simulink model "Copy_5_of_baseModel"  (R2019a)
settings: Solver=ode1  StartTime=0.0  StopTime=2.5  FixedStep=Ts_Power  RelTol=1e-3
PostLoadFcn:
  | %% Init for wind PnO models - global system parameters
  | OVERRIDE_SSN_MEMORY_LIMIT=1;
  | Ts=50e-6;
  | % Ts=50e-10;
  | Ts_Power=Ts;
  | Ts_Control=2*Ts;
  | freq = 50;
  | Fnom=freq;
  | Vac=400e3;
InitFcn:
  | %% Init for wind PnO models - global system parameters
  | OVERRIDE_SSN_MEMORY_LIMIT=1;
  | Ts=50e-6;
  | % Ts=50e-10;
  | Ts_Power=Ts;
  | Ts_Control=2*Ts;
  | freq = 50;
  | Fnom=freq;
  | Vac=225e3;
values from neighbouring files (symbols this model uses):
  ohl_posCap = (0.01e-006)*12    (= 1.2e-07)    [variable.m]
  ohl_posInd = (1.15e-3)/12    (= 9.58333333333e-05)    [variable.m]
  ohl_posR = 0.069/12    (= 0.00575)    [variable.m]
  ohl_zeroCap = (0.004e-006)*12    (= 4.8e-08)    [variable.m]
  ohl_zeroInd = (2.86e-3)/12    (= 0.000238333333333)    [variable.m]
  ohl_zeroR = 0.1725/12    (= 0.014375)    [variable.m]
  sub_posCap = sub_posCap*6    (= 9.6e-07)    [variable.m]
  sub_posInd = sub_posInd/6    (= 0.000233333333333)    [variable.m]
  sub_posR = sub_posR/6    (= 0.006)    [variable.m]
  sub_zeroCap = sub_zeroCap*6    (= 3.84e-07)    [variable.m]
  sub_zeroInd = sub_zeroInd/6    (= 0.000583333333333)    [variable.m]
  sub_zeroR = sub_zeroR/6    (= 0.015)    [variable.m]
  transfo_L1 = 0.05999374    [variable.m]
  transfo_L2 = 0.05999374    [variable.m]
  transfo_R1 = 0.000866667    [variable.m]
  transfo_R2 = 0.00086667    [variable.m]
undefined symbols (not defined in the file or in its folder): D1, D11, Delta, den, DiscIntNeverNeededParam, dx, find_system, gcbh, num, out_Buses, out_WindFarms, sps_rtmsupport
libraries: powerlib x200, simulink x96, powerlib_meascontrol x96, elements x52, eeSinusoidalMeasurement x51, simulink_extras x42, spsVIMeasurementModel x36, eePowerMeasurement x16
(part 12 of 24)

== system Copy_5_of_baseModel/SM_WT1/Impedance Element 1/Impedance Relay Scheme/Fault C-A Measurement ==
  C-A : Inport
  <V : Inport  Port=2
  Complex to Real-Imag : ComplexToRealImag
  Impedance Module : Product  Inputs=*/  SaturateOnIntegerOverflow=on  RndMeth=Zero  InputSameDT=on  OutDataTypeStr=Inherit: Same as first input
  Mux{,1..4} (5 alike) : Mux  Inputs=2
  Voltage Current : Demux  Outputs=2
  Zone 1 : Subsystem  mask(Zone){Xr=ZoneImpedance(1)*sin(LineAngle*pi/180), Rr=ZoneImpedance(1)*cos(LineAngle*pi/180), Td=ZoneTime(1)}
      mask prompts: Xr "Reactance reach [ohm]"; Rr "Resistance reach [ohm]"; Td "Time delay [s]"
  Zone 2 : Subsystem  mask(Zone){Xr=ZoneImpedance(2)*sin(LineAngle*pi/180), Rr=ZoneImpedance(2)*cos(LineAngle*pi/180), Td=ZoneTime(2)}
      mask prompts: Xr "Reactance reach [ohm]"; Rr "Resistance reach [ohm]"; Td "Time delay [s]"
  Zone 3 : Subsystem  mask(Zone){Xr=ZoneImpedance(3)*sin(LineAngle*pi/180), Rr=ZoneImpedance(3)*cos(LineAngle*pi/180), Td=ZoneTime(3)}
      mask prompts: Xr "Reactance reach [ohm]"; Rr "Resistance reach [ohm]"; Td "Time delay [s]"
  Zone 4 : Subsystem  mask(Zone){Xr=ZoneImpedance(4)*sin(LineAngle*pi/180), Rr=ZoneImpedance(4)*cos(LineAngle*pi/180), Td=ZoneTime(4)}
      mask prompts: Xr "Reactance reach [ohm]"; Rr "Resistance reach [ohm]"; Td "Time delay [s]"
  Zone1Z : Terminator
  Zone2Z : Terminator
  Zone3Z : Terminator
  Zone4Z : Terminator
  Zone1 : Outport  InitialOutput=0  VectorParamsAs1DForOutWhenUnconnected=on
  Zone2 : Outport  Port=2  InitialOutput=0  VectorParamsAs1DForOutWhenUnconnected=on
  Zone3 : Outport  Port=3  InitialOutput=0  VectorParamsAs1DForOutWhenUnconnected=on
  Zone4 : Outport  Port=4  InitialOutput=0  VectorParamsAs1DForOutWhenUnconnected=on
  wires:
  Voltage Current/2 -> Impedance Module/2
  Voltage Current/1 -> Impedance Module/1
  Impedance Module/1 -> Complex to Real-Imag/1
  Mux4/1 -> Zone4Z/1
  Mux3/1 -> Zone3Z/1
  Mux2/1 -> Zone2Z/1
  Mux1/1 -> Zone1Z/1
  <V/1 -> Zone 4/2(<V), Zone 3/2(<V), Zone 2/2(<V), Zone 1/2(<V)
  Complex to Real-Imag/2 -> Mux/2
  Complex to Real-Imag/1 -> Mux/1
  Zone 4/1(TRIP) -> Zone4/1
  Zone 3/1(TRIP) -> Zone3/1
  Zone 2/1(TRIP) -> Zone2/1
  Zone 4/3(Zr) -> Mux4/2
  Zone 4/2(Zm) -> Mux4/1
  Zone 3/3(Zr) -> Mux3/2
  Zone 3/2(Zm) -> Mux3/1
  Zone 2/3(Zr) -> Mux2/2
  Zone 2/2(Zm) -> Mux2/1
  Zone 1/3(Zr) -> Mux1/2
  Zone 1/2(Zm) -> Mux1/1
  Zone 1/1(TRIP) -> Zone1/1
  Mux/1 -> Zone 2/1(Z), Zone 4/1(Z), Zone 3/1(Z), Zone 1/1(Z)
  C-A/1 -> Voltage Current/1

== system Copy_5_of_baseModel/SM_WT1/Impedance Element 1/Impedance Relay Scheme/Fault C-G Measurement ==
  C-G : Inport
  <V : Inport  Port=2
  Complex to Real-Imag : ComplexToRealImag
  Impedance Module : Product  Inputs=*/  SaturateOnIntegerOverflow=on  RndMeth=Zero  InputSameDT=on  OutDataTypeStr=Inherit: Same as first input
  Mux{,1..4} (5 alike) : Mux  Inputs=2
  Voltage Current : Demux  Outputs=2
  Zone 1 : Subsystem  mask(Zone){Xr=ZoneImpedance(1)*sin(LineAngle*pi/180), Rr=ZoneImpedance(1)*cos(LineAngle*pi/180), Td=ZoneTime(1)}
      mask prompts: Xr "Reactance reach [ohm]"; Rr "Resistance reach [ohm]"; Td "Time delay [s]"
  Zone 2 : Subsystem  mask(Zone){Xr=ZoneImpedance(2)*sin(LineAngle*pi/180), Rr=ZoneImpedance(2)*cos(LineAngle*pi/180), Td=ZoneTime(2)}
      mask prompts: Xr "Reactance reach [ohm]"; Rr "Resistance reach [ohm]"; Td "Time delay [s]"
  Zone 3 : Subsystem  mask(Zone){Xr=ZoneImpedance(3)*sin(LineAngle*pi/180), Rr=ZoneImpedance(3)*cos(LineAngle*pi/180), Td=ZoneTime(3)}
      mask prompts: Xr "Reactance reach [ohm]"; Rr "Resistance reach [ohm]"; Td "Time delay [s]"
  Zone 4 : Subsystem  mask(Zone){Xr=ZoneImpedance(4)*sin(LineAngle*pi/180), Rr=ZoneImpedance(4)*cos(LineAngle*pi/180), Td=ZoneTime(4)}
      mask prompts: Xr "Reactance reach [ohm]"; Rr "Resistance reach [ohm]"; Td "Time delay [s]"
  Zone1Z : Terminator
  Zone2Z : Terminator
  Zone3Z : Terminator
  Zone4Z : Terminator
  Zone1 : Outport  InitialOutput=0  VectorParamsAs1DForOutWhenUnconnected=on
  Zone2 : Outport  Port=2  InitialOutput=0  VectorParamsAs1DForOutWhenUnconnected=on
  Zone3 : Outport  Port=3  InitialOutput=0  VectorParamsAs1DForOutWhenUnconnected=on
  Zone4 : Outport  Port=4  InitialOutput=0  VectorParamsAs1DForOutWhenUnconnected=on
  wires:
  Voltage Current/2 -> Impedance Module/2
  Voltage Current/1 -> Impedance Module/1
  Impedance Module/1 -> Complex to Real-Imag/1
  Mux4/1 -> Zone4Z/1
  Mux3/1 -> Zone3Z/1
  Mux2/1 -> Zone2Z/1
  Mux1/1 -> Zone1Z/1
  <V/1 -> Zone 4/2(<V), Zone 3/2(<V), Zone 2/2(<V), Zone 1/2(<V)
  Complex to Real-Imag/2 -> Mux/2
  Complex to Real-Imag/1 -> Mux/1
  Zone 4/1(TRIP) -> Zone4/1
  Zone 3/1(TRIP) -> Zone3/1
  Zone 2/1(TRIP) -> Zone2/1
  Zone 4/3(Zr) -> Mux4/2
  Zone 4/2(Zm) -> Mux4/1
  Zone 3/3(Zr) -> Mux3/2
  Zone 3/2(Zm) -> Mux3/1
  Zone 2/3(Zr) -> Mux2/2
  Zone 2/2(Zm) -> Mux2/1
  Zone 1/3(Zr) -> Mux1/2
  Zone 1/2(Zm) -> Mux1/1
  Zone 1/1(TRIP) -> Zone1/1
  Mux/1 -> Zone 2/1(Z), Zone 4/1(Z), Zone 3/1(Z), Zone 1/1(Z)
  C-G/1 -> Voltage Current/1

== system Copy_5_of_baseModel/SM_WT1/Impedance Element 1/Impedance Relay Scheme/Logic Matrix ==
  note: Impedance Relay - Logic Signal Matrix
  A-G : Inport
  B-G : Inport  Port=2
  C-G : Inport  Port=3
  B-C : Inport  Port=4
  C-A : Inport  Port=5
  A-B-C : Inport  Port=6
  A : Logic  Operator=OR  Inputs=3
  A-B-C1 : Logic  Operator=OR  Inputs=4
  "A-G1 " : Logic  Operator=OR  Inputs=4
  B : Logic  Operator=OR  Inputs=3
  B-C1 : Logic  Operator=OR  Inputs=4
  B-G1 : Logic  Operator=OR  Inputs=4
  C : Logic  Operator=OR  Inputs=4
  C-A1 : Logic  Operator=OR  Inputs=4
  C-G1 : Logic  Operator=OR  Inputs=4
  Demux{,1..5} (6 alike) : Demux
  G : Logic  Operator=OR  Inputs=3
  Mux5 : Mux
  zone{1..4} (4 alike) : Logic  Operator=OR  Inputs=6
  " Zone1" : Outport  InitialOutput=0  VectorParamsAs1DForOutWhenUnconnected=on
  " Zone2" : Outport  Port=2  InitialOutput=0  VectorParamsAs1DForOutWhenUnconnected=on
  " Zone3" : Outport  Port=3  InitialOutput=0  VectorParamsAs1DForOutWhenUnconnected=on
  " Zone4" : Outport  Port=4  InitialOutput=0  VectorParamsAs1DForOutWhenUnconnected=on
  Fault Type : Outport  Port=5  InitialOutput=0  VectorParamsAs1DForOutWhenUnconnected=on
  wires:
  G/1 -> Mux5/4
  C/1 -> Mux5/3
  B/1 -> Mux5/2
  A/1 -> Mux5/1
  B-G1/1 -> G/2, B/1
  C-G1/1 -> G/1, C/1
  B-C1/1 -> C/2, B/2
  A-B-C1/1 -> B/3, A/3, C/4
  C-A1/1 -> A/2, C/3
  "A-G1 "/1 -> G/3, A/1
  Demux5/4 -> A-B-C1/4, zone4/6
  Demux5/3 -> A-B-C1/3, zone3/6
  Demux5/2 -> A-B-C1/2, zone2/6
  Demux5/1 -> A-B-C1/1, zone1/6
  Demux4/4 -> C-A1/4, zone4/5
  Demux4/3 -> C-A1/3, zone3/5
  Demux4/2 -> C-A1/2, zone2/5
  Demux4/1 -> C-A1/1, zone1/5
  Demux3/4 -> B-C1/4, zone4/4
  Demux3/3 -> B-C1/3, zone3/4
  Demux3/2 -> B-C1/2, zone2/4
  Demux3/1 -> B-C1/1, zone1/4
  Demux2/4 -> C-G1/4, zone4/3
  Demux2/3 -> C-G1/3, zone3/3
  Demux2/2 -> C-G1/2, zone2/3
  Demux2/1 -> C-G1/1, zone1/3
  Demux1/4 -> B-G1/4, zone4/2
  Demux1/3 -> B-G1/3, zone3/2
  Demux1/2 -> B-G1/2, zone2/2
  Demux1/1 -> B-G1/1, zone1/2
  Demux/4 -> "A-G1 "/4, zone4/1
  Demux/3 -> "A-G1 "/3, zone3/1
  Demux/2 -> "A-G1 "/2, zone2/1
  Demux/1 -> "A-G1 "/1, zone1/1
  A-G/1 -> Demux/1
  B-G/1 -> Demux1/1
  A-B-C/1 -> Demux5/1
  C-A/1 -> Demux4/1
  B-C/1 -> Demux3/1
  C-G/1 -> Demux2/1
  Mux5/1 -> Fault Type/1
  zone1/1 -> " Zone1"/1
  zone2/1 -> " Zone2"/1
  zone4/1 -> " Zone4"/1
  zone3/1 -> " Zone3"/1

== system Copy_5_of_baseModel/SM_WT1/Impedance Element 1/Impedance Relay Scheme/Tripping Logic ==
  note: Impedance Relay - Tripping Logic
  zone1 : Inport
  zone2 : Inport  Port=2
  zone3 : Inport  Port=3
  zone4 : Inport  Port=4
  <V : Inport  Port=5
  Add{,1..3} (4 alike) : Sum
  Constant : Constant  Value=2
  Mux : Mux  Inputs=5
  Mux6 : Mux
  ZM1 + ZM2*t2 + ZM3*t3 + ZM4*t4 : Logic  Operator=OR  Inputs=4
  x2 : Gain  Gain=2  SaturateOnIntegerOverflow=on  OutDataTypeStr=Inherit: Same as input  ParamDataTypeStr=Inherit: Same as input
  x3 : Gain  Gain=3  SaturateOnIntegerOverflow=on  OutDataTypeStr=Inherit: Same as input  ParamDataTypeStr=Inherit: Same as input
  x4 : Gain  Gain=4  SaturateOnIntegerOverflow=on  OutDataTypeStr=Inherit: Same as input  ParamDataTypeStr=Inherit: Same as input
  TRIP : Outport  InitialOutput=0  VectorParamsAs1DForOutWhenUnconnected=on
  Logic Signals : Outport  Port=2  InitialOutput=0  VectorParamsAs1DForOutWhenUnconnected=on
  Fault Zone : Outport  Port=3  InitialOutput=0  VectorParamsAs1DForOutWhenUnconnected=on
  wires:
  Mux6/1 -> Fault Zone/1
  x3/1 -> Add2/2
  x4/1 -> Add3/2
  x2/1 -> Add1/2
  Constant/1 -> x4/1, x3/1, x2/1, Add/2
  Add3/1 -> Mux/5
  Add2/1 -> Mux/4
  Add1/1 -> Mux/3
  Add/1 -> Mux/2
  zone4/1 -> Mux6/4, Add3/1, ZM1 + ZM2*t2 + ZM3*t3 + ZM4*t4/4
  zone3/1 -> Mux6/3, Add2/1, ZM1 + ZM2*t2 + ZM3*t3 + ZM4*t4/3
  zone2/1 -> Add1/1, Mux6/2, ZM1 + ZM2*t2 + ZM3*t3 + ZM4*t4/2
  zone1/1 -> Mux6/1, Add/1, ZM1 + ZM2*t2 + ZM3*t3 + ZM4*t4/1
  ZM1 + ZM2*t2 + ZM3*t3 + ZM4*t4/1 -> TRIP/1
  Mux/1 -> Logic Signals/1
  <V/1 -> Mux/1

== system Copy_5_of_baseModel/SM_WT1/Impedance Element 1/Impedance Relay Scheme/Undervoltage ==
  "Vabc  " : Inport
  Abs : Abs
  Abs1 : Abs
  Abs2 : Abs
  Demux2 : Demux  Outputs=3
  Logical Operator : Logic  Operator=OR  Inputs=3
  Relational Operator : RelationalOperator  Operator=<  RndMeth=Nearest  InputSameDT=on
  Relational Operator1 : RelationalOperator  Operator=<  RndMeth=Nearest  InputSameDT=on
  Relational Operator2 : RelationalOperator  Operator=<  RndMeth=Nearest  InputSameDT=on
  underV Threshold : Constant  Value=underV
  <V : Outport  InitialOutput=0  VectorParamsAs1DForOutWhenUnconnected=on
  wires:
  Demux2/3 -> Abs2/1
  Demux2/2 -> Abs1/1
  Abs1/1 -> Relational Operator2/1
  Abs2/1 -> Relational Operator1/1
  Demux2/1 -> Abs/1
  Abs/1 -> Relational Operator/1
  Relational Operator1/1 -> Logical Operator/3
  Relational Operator/1 -> Logical Operator/1
  Relational Operator2/1 -> Logical Operator/2
  Logical Operator/1 -> <V/1
  underV Threshold/1 -> Relational Operator1/2, Relational Operator2/2, Relational Operator/2
  "Vabc  "/1 -> Demux2/1

== system Copy_5_of_baseModel/SM_WT1/Impedance Element 2/Impedance Relay Scheme/Analog filtering, signal conditioning ==
  note: Acquisition Block- analog filtering,
      | signal conditioning, sampling.
  Vin : Inport
  Iin : Inport  Port=2
  CURRENTS : Subsystem
  Mux{1..4} (4 alike) : Mux  Inputs=3
  VOLTAGES : Subsystem
  Vf : Outport  InitialOutput=0  VectorParamsAs1DForOutWhenUnconnected=on
  If : Outport  Port=2  InitialOutput=0  VectorParamsAs1DForOutWhenUnconnected=on
  If0 : Outport  Port=3  InitialOutput=0  VectorParamsAs1DForOutWhenUnconnected=on
  vf : Outport  Port=4  InitialOutput=0  VectorParamsAs1DForOutWhenUnconnected=on
  if : Outport  Port=5  InitialOutput=0  VectorParamsAs1DForOutWhenUnconnected=on
  wires:
  CURRENTS/4(k0I0f) -> If0/1
  Mux4/1 -> if/1
  Mux3/1 -> If/1
  CURRENTS/7(icf) -> Mux4/3
  CURRENTS/6(ibf) -> Mux4/2
  CURRENTS/5(iaf) -> Mux4/1
  CURRENTS/3(ICf) -> Mux3/3
  CURRENTS/2(IBf) -> Mux3/2
  CURRENTS/1(IAf) -> Mux3/1
  Iin/1 -> CURRENTS/1(Iabc)
  Mux2/1 -> vf/1
  VOLTAGES/6(vcf) -> Mux2/3
  VOLTAGES/5(vbf) -> Mux2/2
  VOLTAGES/4(vaf) -> Mux2/1
  VOLTAGES/3(VCf) -> Mux1/3
  VOLTAGES/2(VBf) -> Mux1/2
  VOLTAGES/1(VAf) -> Mux1/1
  Vin/1 -> VOLTAGES/1(Vabc)
  Mux1/1 -> Vf/1

== system Copy_5_of_baseModel/SM_WT1/Impedance Element 2/Impedance Relay Scheme/Combination of Voltages and Currents into 6 pairs (for each type of fault) ==
  note: Voltage and current combination block
  Vf : Inport
  If : Inport  Port=2
  If0 : Inport  Port=3
  "Currents Ia, Ib, Ic, kIo" : Demux  Outputs=3
  Ia+kIo : Sum  SaturateOnIntegerOverflow=on  InputSameDT=on  OutDataTypeStr=Inherit: Same as first input
  Ia-Ib : Sum  Inputs=+-  SaturateOnIntegerOverflow=on  InputSameDT=on  OutDataTypeStr=Inherit: Same as first input
  Ib+kIo : Sum  SaturateOnIntegerOverflow=on  InputSameDT=on  OutDataTypeStr=Inherit: Same as first input
  Ib-Ic : Sum  Inputs=+-  SaturateOnIntegerOverflow=on  InputSameDT=on  OutDataTypeStr=Inherit: Same as first input
  Ic+kIo : Sum  SaturateOnIntegerOverflow=on  InputSameDT=on  OutDataTypeStr=Inherit: Same as first input
  Ic-Ia : Sum  Inputs=+-  SaturateOnIntegerOverflow=on  InputSameDT=on  OutDataTypeStr=Inherit: Same as first input
  Mux{10..15} (6 alike) : Mux  Inputs=2
  Va-Vb : Sum  Inputs=+-  SaturateOnIntegerOverflow=on  InputSameDT=on  OutDataTypeStr=Inherit: Same as first input
  Vb-Vc : Sum  Inputs=+-  SaturateOnIntegerOverflow=on  InputSameDT=on  OutDataTypeStr=Inherit: Same as first input
  Vc-Va : Sum  Inputs=+-  SaturateOnIntegerOverflow=on  InputSameDT=on  OutDataTypeStr=Inherit: Same as first input
  "Voltages Va,Vb, Vc" : Demux  Outputs=3
  "Volt, Curr A-G" : Outport  InitialOutput=0  VectorParamsAs1DForOutWhenUnconnected=on
  "Volt, Curr B-G" : Outport  Port=2  InitialOutput=0  VectorParamsAs1DForOutWhenUnconnected=on
  "Volt, Curr C-G" : Outport  Port=3  InitialOutput=0  VectorParamsAs1DForOutWhenUnconnected=on
  "Volt, Curr B-C,B-C-G" : Outport  Port=4  InitialOutput=0  VectorParamsAs1DForOutWhenUnconnected=on
  "Volt, Curr C-A,C-A-G" : Outport  Port=5  InitialOutput=0  VectorParamsAs1DForOutWhenUnconnected=on
  "Volt, Curr A-B,A-B-C-G" : Outport  Port=6  InitialOutput=0  VectorParamsAs1DForOutWhenUnconnected=on
  wires:
  If0/1 -> Ib+kIo/2, Ia+kIo/2, Ic+kIo/2
  Mux13/1 -> "Volt, Curr B-C,B-C-G"/1
  Vb-Vc/1 -> Mux13/1
  Ib-Ic/1 -> Mux13/2
  Mux12/1 -> "Volt, Curr C-G"/1
  Ic+kIo/1 -> Mux12/2
  If/1 -> "Currents Ia, Ib, Ic, kIo"/1
  "Voltages Va,Vb, Vc"/3 -> Vc-Va/1, Vb-Vc/2, Mux12/1
  "Voltages Va,Vb, Vc"/2 -> Vb-Vc/1, Mux11/1, Va-Vb/2
  "Voltages Va,Vb, Vc"/1 -> Va-Vb/1, Mux10/1, Vc-Va/2
  Vf/1 -> "Voltages Va,Vb, Vc"/1
  Mux15/1 -> "Volt, Curr A-B,A-B-C-G"/1
  Mux14/1 -> "Volt, Curr C-A,C-A-G"/1
  Vc-Va/1 -> Mux14/1
  Mux11/1 -> "Volt, Curr B-G"/1
  Mux10/1 -> "Volt, Curr A-G"/1
  Ia+kIo/1 -> Mux10/2
  Ib+kIo/1 -> Mux11/2
  Ic-Ia/1 -> Mux14/2
  Va-Vb/1 -> Mux15/1
  Ia-Ib/1 -> Mux15/2
  "Currents Ia, Ib, Ic, kIo"/2 -> Ia-Ib/2, Ib-Ic/1, Ib+kIo/1
  "Currents Ia, Ib, Ic, kIo"/3 -> Ic-Ia/1, Ib-Ic/2, Ic+kIo/1
  "Currents Ia, Ib, Ic, kIo"/1 -> Ia-Ib/1, Ic-Ia/2, Ia+kIo/1

== system Copy_5_of_baseModel/SM_WT1/Impedance Element 2/Impedance Relay Scheme/Fault A-B-C Measurement ==
  A-B-C : Inport
  <V : Inport  Port=2
  Complex to Real-Imag : ComplexToRealImag
  Impedance Module : Product  Inputs=*/  SaturateOnIntegerOverflow=on  RndMeth=Zero  InputSameDT=on  OutDataTypeStr=Inherit: Same as first input
  Mux{,1..4} (5 alike) : Mux  Inputs=2
  Voltage Current : Demux  Outputs=2
  Zone 1 : Subsystem  mask(Zone){Xr=ZoneImpedance(1)*sin(LineAngle*pi/180), Rr=ZoneImpedance(1)*cos(LineAngle*pi/180), Td=ZoneTime(1)}
      mask prompts: Xr "Reactance reach [ohm]"; Rr "Resistance reach [ohm]"; Td "Time delay [s]"
  Zone 2 : Subsystem  mask(Zone){Xr=ZoneImpedance(2)*sin(LineAngle*pi/180), Rr=ZoneImpedance(2)*cos(LineAngle*pi/180), Td=ZoneTime(2)}
      mask prompts: Xr "Reactance reach [ohm]"; Rr "Resistance reach [ohm]"; Td "Time delay [s]"
  Zone 3 : Subsystem  mask(Zone){Xr=ZoneImpedance(3)*sin(LineAngle*pi/180), Rr=ZoneImpedance(3)*cos(LineAngle*pi/180), Td=ZoneTime(3)}
      mask prompts: Xr "Reactance reach [ohm]"; Rr "Resistance reach [ohm]"; Td "Time delay [s]"
  Zone 4 : Subsystem  mask(Zone){Xr=ZoneImpedance(4)*sin(LineAngle*pi/180), Rr=ZoneImpedance(4)*cos(LineAngle*pi/180), Td=ZoneTime(4)}
      mask prompts: Xr "Reactance reach [ohm]"; Rr "Resistance reach [ohm]"; Td "Time delay [s]"
  Zone1Z : Terminator
  Zone2Z : Terminator
  Zone3Z : Terminator
  Zone4Z : Terminator
  Zone1 : Outport  InitialOutput=0  VectorParamsAs1DForOutWhenUnconnected=on
  Zone2 : Outport  Port=2  InitialOutput=0  VectorParamsAs1DForOutWhenUnconnected=on
  Zone3 : Outport  Port=3  InitialOutput=0  VectorParamsAs1DForOutWhenUnconnected=on
  Zone4 : Outport  Port=4  InitialOutput=0  VectorParamsAs1DForOutWhenUnconnected=on
  wires:
  A-B-C/1 -> Voltage Current/1
  Mux/1 -> Zone 1/1(Z), Zone 3/1(Z), Zone 4/1(Z), Zone 2/1(Z)
  Zone 1/1(TRIP) -> Zone1/1
  Zone 1/2(Zm) -> Mux1/1
  Zone 1/3(Zr) -> Mux1/2
  Zone 2/2(Zm) -> Mux2/1
  Zone 2/3(Zr) -> Mux2/2
  Zone 3/2(Zm) -> Mux3/1
  Zone 3/3(Zr) -> Mux3/2
  Zone 4/2(Zm) -> Mux4/1
  Zone 4/3(Zr) -> Mux4/2
  Zone 2/1(TRIP) -> Zone2/1
  Zone 3/1(TRIP) -> Zone3/1
  Zone 4/1(TRIP) -> Zone4/1
  Complex to Real-Imag/1 -> Mux/1
  Complex to Real-Imag/2 -> Mux/2
  <V/1 -> Zone 1/2(<V), Zone 2/2(<V), Zone 3/2(<V), Zone 4/2(<V)
  Mux1/1 -> Zone1Z/1
  Mux2/1 -> Zone2Z/1
  Mux3/1 -> Zone3Z/1
  Mux4/1 -> Zone4Z/1
  Impedance Module/1 -> Complex to Real-Imag/1
  Voltage Current/1 -> Impedance Module/1
  Voltage Current/2 -> Impedance Module/2

== system Copy_5_of_baseModel/SM_WT1/Impedance Element 2/Impedance Relay Scheme/Fault A-G Measurement ==
  A-G : Inport
  <V : Inport  Port=2
  Complex to Real-Imag : ComplexToRealImag
  Impedance Module : Product  Inputs=*/  SaturateOnIntegerOverflow=on  RndMeth=Zero  InputSameDT=on  OutDataTypeStr=Inherit: Same as first input
  Mux{,1..4} (5 alike) : Mux  Inputs=2
  Voltage Current : Demux  Outputs=2
  Zone 1 : Subsystem  mask(Zone){Xr=ZoneImpedance(1)*sin(LineAngle*pi/180), Rr=ZoneImpedance(1)*cos(LineAngle*pi/180), Td=ZoneTime(1)}
      mask prompts: Xr "Reactance reach [ohm]"; Rr "Resistance reach [ohm]"; Td "Time delay [s]"
  Zone 2 : Subsystem  mask(Zone){Xr=ZoneImpedance(2)*sin(LineAngle*pi/180), Rr=ZoneImpedance(2)*cos(LineAngle*pi/180), Td=ZoneTime(2)}
      mask prompts: Xr "Reactance reach [ohm]"; Rr "Resistance reach [ohm]"; Td "Time delay [s]"
  Zone 3 : Subsystem  mask(Zone){Xr=ZoneImpedance(3)*sin(LineAngle*pi/180), Rr=ZoneImpedance(3)*cos(LineAngle*pi/180), Td=ZoneTime(3)}
      mask prompts: Xr "Reactance reach [ohm]"; Rr "Resistance reach [ohm]"; Td "Time delay [s]"
  Zone 4 : Subsystem  mask(Zone){Xr=ZoneImpedance(4)*sin(LineAngle*pi/180), Rr=ZoneImpedance(4)*cos(LineAngle*pi/180), Td=ZoneTime(4)}
      mask prompts: Xr "Reactance reach [ohm]"; Rr "Resistance reach [ohm]"; Td "Time delay [s]"
  Zone1Z : Terminator
  Zone2Z : Terminator
  Zone3Z : Terminator
  Zone4Z : Terminator
  Zone1 : Outport  InitialOutput=0  VectorParamsAs1DForOutWhenUnconnected=on
  Zone2 : Outport  Port=2  InitialOutput=0  VectorParamsAs1DForOutWhenUnconnected=on
  Zone3 : Outport  Port=3  InitialOutput=0  VectorParamsAs1DForOutWhenUnconnected=on
  Zone4 : Outport  Port=4  InitialOutput=0  VectorParamsAs1DForOutWhenUnconnected=on
  wires:
  Voltage Current/2 -> Impedance Module/2
  Voltage Current/1 -> Impedance Module/1
  Impedance Module/1 -> Complex to Real-Imag/1
  Mux4/1 -> Zone4Z/1
  Mux3/1 -> Zone3Z/1
  Mux2/1 -> Zone2Z/1
  Mux1/1 -> Zone1Z/1
  <V/1 -> Zone 4/2(<V), Zone 3/2(<V), Zone 2/2(<V), Zone 1/2(<V)
  Complex to Real-Imag/2 -> Mux/2
  Complex to Real-Imag/1 -> Mux/1
  Zone 4/1(TRIP) -> Zone4/1
  Zone 3/1(TRIP) -> Zone3/1
  Zone 2/1(TRIP) -> Zone2/1
  Zone 4/3(Zr) -> Mux4/2
  Zone 4/2(Zm) -> Mux4/1
  Zone 3/3(Zr) -> Mux3/2
  Zone 3/2(Zm) -> Mux3/1
  Zone 2/3(Zr) -> Mux2/2
  Zone 2/2(Zm) -> Mux2/1
  Zone 1/3(Zr) -> Mux1/2
  Zone 1/2(Zm) -> Mux1/1
  Zone 1/1(TRIP) -> Zone1/1
  Mux/1 -> Zone 2/1(Z), Zone 4/1(Z), Zone 3/1(Z), Zone 1/1(Z)
  A-G/1 -> Voltage Current/1

== system Copy_5_of_baseModel/SM_WT1/Impedance Element 2/Impedance Relay Scheme/Fault B-C Measurement ==
  B-C : Inport
  <V : Inport  Port=2
  Complex to Real-Imag : ComplexToRealImag
  Impedance Module : Product  Inputs=*/  SaturateOnIntegerOverflow=on  RndMeth=Zero  InputSameDT=on  OutDataTypeStr=Inherit: Same as first input
  Mux{,1..4} (5 alike) : Mux  Inputs=2
  Voltage Current : Demux  Outputs=2
  Zone 1 : Subsystem  mask(Zone){Xr=ZoneImpedance(1)*sin(LineAngle*pi/180), Rr=ZoneImpedance(1)*cos(LineAngle*pi/180), Td=ZoneTime(1)}
      mask prompts: Xr "Reactance reach [ohm]"; Rr "Resistance reach [ohm]"; Td "Time delay [s]"
  Zone 2 : Subsystem  mask(Zone){Xr=ZoneImpedance(2)*sin(LineAngle*pi/180), Rr=ZoneImpedance(2)*cos(LineAngle*pi/180), Td=ZoneTime(2)}
      mask prompts: Xr "Reactance reach [ohm]"; Rr "Resistance reach [ohm]"; Td "Time delay [s]"
  Zone 3 : Subsystem  mask(Zone){Xr=ZoneImpedance(3)*sin(LineAngle*pi/180), Rr=ZoneImpedance(3)*cos(LineAngle*pi/180), Td=ZoneTime(3)}
      mask prompts: Xr "Reactance reach [ohm]"; Rr "Resistance reach [ohm]"; Td "Time delay [s]"
  Zone 4 : Subsystem  mask(Zone){Xr=ZoneImpedance(4)*sin(LineAngle*pi/180), Rr=ZoneImpedance(4)*cos(LineAngle*pi/180), Td=ZoneTime(4)}
      mask prompts: Xr "Reactance reach [ohm]"; Rr "Resistance reach [ohm]"; Td "Time delay [s]"
  Zone1Z : Terminator
  Zone2Z : Terminator
  Zone3Z : Terminator
  Zone4Z : Terminator
  Zone1 : Outport  InitialOutput=0  VectorParamsAs1DForOutWhenUnconnected=on
  Zone2 : Outport  Port=2  InitialOutput=0  VectorParamsAs1DForOutWhenUnconnected=on
  Zone3 : Outport  Port=3  InitialOutput=0  VectorParamsAs1DForOutWhenUnconnected=on
  Zone4 : Outport  Port=4  InitialOutput=0  VectorParamsAs1DForOutWhenUnconnected=on
  wires:
  B-C/1 -> Voltage Current/1
  Mux/1 -> Zone 1/1(Z), Zone 3/1(Z), Zone 4/1(Z), Zone 2/1(Z)
  Zone 1/1(TRIP) -> Zone1/1
  Zone 1/2(Zm) -> Mux1/1
  Zone 1/3(Zr) -> Mux1/2
  Zone 2/2(Zm) -> Mux2/1
  Zone 2/3(Zr) -> Mux2/2
  Zone 3/2(Zm) -> Mux3/1
  Zone 3/3(Zr) -> Mux3/2
  Zone 4/2(Zm) -> Mux4/1
  Zone 4/3(Zr) -> Mux4/2
  Zone 2/1(TRIP) -> Zone2/1
  Zone 3/1(TRIP) -> Zone3/1
  Zone 4/1(TRIP) -> Zone4/1
  Complex to Real-Imag/1 -> Mux/1
  Complex to Real-Imag/2 -> Mux/2
  <V/1 -> Zone 1/2(<V), Zone 2/2(<V), Zone 3/2(<V), Zone 4/2(<V)
  Mux1/1 -> Zone1Z/1
  Mux2/1 -> Zone2Z/1
  Mux3/1 -> Zone3Z/1
  Mux4/1 -> Zone4Z/1
  Impedance Module/1 -> Complex to Real-Imag/1
  Voltage Current/1 -> Impedance Module/1
  Voltage Current/2 -> Impedance Module/2

== system Copy_5_of_baseModel/SM_WT1/Impedance Element 2/Impedance Relay Scheme/Fault B-G Measurement ==
  B-G : Inport
  <V : Inport  Port=2
  Complex to Real-Imag : ComplexToRealImag
  Impedance Module : Product  Inputs=*/  SaturateOnIntegerOverflow=on  RndMeth=Zero  InputSameDT=on  OutDataTypeStr=Inherit: Same as first input
  Mux{,1..4} (5 alike) : Mux  Inputs=2
  Voltage Current : Demux  Outputs=2
  Zone 1 : Subsystem  mask(Zone){Xr=ZoneImpedance(1)*sin(LineAngle*pi/180), Rr=ZoneImpedance(1)*cos(LineAngle*pi/180), Td=ZoneTime(1)}
      mask prompts: Xr "Reactance reach [ohm]"; Rr "Resistance reach [ohm]"; Td "Time delay [s]"
  Zone 2 : Subsystem  mask(Zone){Xr=ZoneImpedance(2)*sin(LineAngle*pi/180), Rr=ZoneImpedance(2)*cos(LineAngle*pi/180), Td=ZoneTime(2)}
      mask prompts: Xr "Reactance reach [ohm]"; Rr "Resistance reach [ohm]"; Td "Time delay [s]"
  Zone 3 : Subsystem  mask(Zone){Xr=ZoneImpedance(3)*sin(LineAngle*pi/180), Rr=ZoneImpedance(3)*cos(LineAngle*pi/180), Td=ZoneTime(3)}
      mask prompts: Xr "Reactance reach [ohm]"; Rr "Resistance reach [ohm]"; Td "Time delay [s]"
  Zone 4 : Subsystem  mask(Zone){Xr=ZoneImpedance(4)*sin(LineAngle*pi/180), Rr=ZoneImpedance(4)*cos(LineAngle*pi/180), Td=ZoneTime(4)}
      mask prompts: Xr "Reactance reach [ohm]"; Rr "Resistance reach [ohm]"; Td "Time delay [s]"
  Zone1Z : Terminator
  Zone2Z : Terminator
  Zone3Z : Terminator
  Zone4Z : Terminator
  Zone1 : Outport  InitialOutput=0  VectorParamsAs1DForOutWhenUnconnected=on
  Zone2 : Outport  Port=2  InitialOutput=0  VectorParamsAs1DForOutWhenUnconnected=on
  Zone3 : Outport  Port=3  InitialOutput=0  VectorParamsAs1DForOutWhenUnconnected=on
  Zone4 : Outport  Port=4  InitialOutput=0  VectorParamsAs1DForOutWhenUnconnected=on
  wires:
  B-G/1 -> Voltage Current/1
  Mux/1 -> Zone 1/1(Z), Zone 3/1(Z), Zone 4/1(Z), Zone 2/1(Z)
  Zone 1/1(TRIP) -> Zone1/1
  Zone 1/2(Zm) -> Mux1/1
  Zone 1/3(Zr) -> Mux1/2
  Zone 2/2(Zm) -> Mux2/1
  Zone 2/3(Zr) -> Mux2/2
  Zone 3/2(Zm) -> Mux3/1
  Zone 3/3(Zr) -> Mux3/2
  Zone 4/2(Zm) -> Mux4/1
  Zone 4/3(Zr) -> Mux4/2
  Zone 2/1(TRIP) -> Zone2/1
  Zone 3/1(TRIP) -> Zone3/1
  Zone 4/1(TRIP) -> Zone4/1
  Complex to Real-Imag/1 -> Mux/1
  Complex to Real-Imag/2 -> Mux/2
  <V/1 -> Zone 1/2(<V), Zone 2/2(<V), Zone 3/2(<V), Zone 4/2(<V)
  Mux1/1 -> Zone1Z/1
  Mux2/1 -> Zone2Z/1
  Mux3/1 -> Zone3Z/1
  Mux4/1 -> Zone4Z/1
  Impedance Module/1 -> Complex to Real-Imag/1
  Voltage Current/1 -> Impedance Module/1
  Voltage Current/2 -> Impedance Module/2

== system Copy_5_of_baseModel/SM_WT1/Impedance Element 2/Impedance Relay Scheme/Fault C-A Measurement ==
  C-A : Inport
  <V : Inport  Port=2
  Complex to Real-Imag : ComplexToRealImag
  Impedance Module : Product  Inputs=*/  SaturateOnIntegerOverflow=on  RndMeth=Zero  InputSameDT=on  OutDataTypeStr=Inherit: Same as first input
  Mux{,1..4} (5 alike) : Mux  Inputs=2
  Voltage Current : Demux  Outputs=2
  Zone 1 : Subsystem  mask(Zone){Xr=ZoneImpedance(1)*sin(LineAngle*pi/180), Rr=ZoneImpedance(1)*cos(LineAngle*pi/180), Td=ZoneTime(1)}
      mask prompts: Xr "Reactance reach [ohm]"; Rr "Resistance reach [ohm]"; Td "Time delay [s]"
  Zone 2 : Subsystem  mask(Zone){Xr=ZoneImpedance(2)*sin(LineAngle*pi/180), Rr=ZoneImpedance(2)*cos(LineAngle*pi/180), Td=ZoneTime(2)}
      mask prompts: Xr "Reactance reach [ohm]"; Rr "Resistance reach [ohm]"; Td "Time delay [s]"
  Zone 3 : Subsystem  mask(Zone){Xr=ZoneImpedance(3)*sin(LineAngle*pi/180), Rr=ZoneImpedance(3)*cos(LineAngle*pi/180), Td=ZoneTime(3)}
      mask prompts: Xr "Reactance reach [ohm]"; Rr "Resistance reach [ohm]"; Td "Time delay [s]"
  Zone 4 : Subsystem  mask(Zone){Xr=ZoneImpedance(4)*sin(LineAngle*pi/180), Rr=ZoneImpedance(4)*cos(LineAngle*pi/180), Td=ZoneTime(4)}
      mask prompts: Xr "Reactance reach [ohm]"; Rr "Resistance reach [ohm]"; Td "Time delay [s]"
  Zone1Z : Terminator
  Zone2Z : Terminator
  Zone3Z : Terminator
  Zone4Z : Terminator
  Zone1 : Outport  InitialOutput=0  VectorParamsAs1DForOutWhenUnconnected=on
  Zone2 : Outport  Port=2  InitialOutput=0  VectorParamsAs1DForOutWhenUnconnected=on
  Zone3 : Outport  Port=3  InitialOutput=0  VectorParamsAs1DForOutWhenUnconnected=on
  Zone4 : Outport  Port=4  InitialOutput=0  VectorParamsAs1DForOutWhenUnconnected=on
  wires:
  Voltage Current/2 -> Impedance Module/2
  Voltage Current/1 -> Impedance Module/1
  Impedance Module/1 -> Complex to Real-Imag/1
  Mux4/1 -> Zone4Z/1
  Mux3/1 -> Zone3Z/1
  Mux2/1 -> Zone2Z/1
  Mux1/1 -> Zone1Z/1
  <V/1 -> Zone 4/2(<V), Zone 3/2(<V), Zone 2/2(<V), Zone 1/2(<V)
  Complex to Real-Imag/2 -> Mux/2
  Complex to Real-Imag/1 -> Mux/1
  Zone 4/1(TRIP) -> Zone4/1
  Zone 3/1(TRIP) -> Zone3/1
  Zone 2/1(TRIP) -> Zone2/1
  Zone 4/3(Zr) -> Mux4/2
  Zone 4/2(Zm) -> Mux4/1
  Zone 3/3(Zr) -> Mux3/2
  Zone 3/2(Zm) -> Mux3/1
  Zone 2/3(Zr) -> Mux2/2
  Zone 2/2(Zm) -> Mux2/1
  Zone 1/3(Zr) -> Mux1/2
  Zone 1/2(Zm) -> Mux1/1
  Zone 1/1(TRIP) -> Zone1/1
  Mux/1 -> Zone 2/1(Z), Zone 4/1(Z), Zone 3/1(Z), Zone 1/1(Z)
  C-A/1 -> Voltage Current/1

== system Copy_5_of_baseModel/SM_WT1/Impedance Element 2/Impedance Relay Scheme/Fault C-G Measurement ==
  C-G : Inport
  <V : Inport  Port=2
  Complex to Real-Imag : ComplexToRealImag
  Impedance Module : Product  Inputs=*/  SaturateOnIntegerOverflow=on  RndMeth=Zero  InputSameDT=on  OutDataTypeStr=Inherit: Same as first input
  Mux{,1..4} (5 alike) : Mux  Inputs=2
  Voltage Current : Demux  Outputs=2
  Zone 1 : Subsystem  mask(Zone){Xr=ZoneImpedance(1)*sin(LineAngle*pi/180), Rr=ZoneImpedance(1)*cos(LineAngle*pi/180), Td=ZoneTime(1)}
      mask prompts: Xr "Reactance reach [ohm]"; Rr "Resistance reach [ohm]"; Td "Time delay [s]"
  Zone 2 : Subsystem  mask(Zone){Xr=ZoneImpedance(2)*sin(LineAngle*pi/180), Rr=ZoneImpedance(2)*cos(LineAngle*pi/180), Td=ZoneTime(2)}
      mask prompts: Xr "Reactance reach [ohm]"; Rr "Resistance reach [ohm]"; Td "Time delay [s]"
  Zone 3 : Subsystem  mask(Zone){Xr=ZoneImpedance(3)*sin(LineAngle*pi/180), Rr=ZoneImpedance(3)*cos(LineAngle*pi/180), Td=ZoneTime(3)}
      mask prompts: Xr "Reactance reach [ohm]"; Rr "Resistance reach [ohm]"; Td "Time delay [s]"
  Zone 4 : Subsystem  mask(Zone){Xr=ZoneImpedance(4)*sin(LineAngle*pi/180), Rr=ZoneImpedance(4)*cos(LineAngle*pi/180), Td=ZoneTime(4)}
      mask prompts: Xr "Reactance reach [ohm]"; Rr "Resistance reach [ohm]"; Td "Time delay [s]"
  Zone1Z : Terminator
  Zone2Z : Terminator
  Zone3Z : Terminator
  Zone4Z : Terminator
  Zone1 : Outport  InitialOutput=0  VectorParamsAs1DForOutWhenUnconnected=on
  Zone2 : Outport  Port=2  InitialOutput=0  VectorParamsAs1DForOutWhenUnconnected=on
  Zone3 : Outport  Port=3  InitialOutput=0  VectorParamsAs1DForOutWhenUnconnected=on
  Zone4 : Outport  Port=4  InitialOutput=0  VectorParamsAs1DForOutWhenUnconnected=on
  wires:
  Voltage Current/2 -> Impedance Module/2
  Voltage Current/1 -> Impedance Module/1
  Impedance Module/1 -> Complex to Real-Imag/1
  Mux4/1 -> Zone4Z/1
  Mux3/1 -> Zone3Z/1
  Mux2/1 -> Zone2Z/1
  Mux1/1 -> Zone1Z/1
  <V/1 -> Zone 4/2(<V), Zone 3/2(<V), Zone 2/2(<V), Zone 1/2(<V)
  Complex to Real-Imag/2 -> Mux/2
  Complex to Real-Imag/1 -> Mux/1
  Zone 4/1(TRIP) -> Zone4/1
  Zone 3/1(TRIP) -> Zone3/1
  Zone 2/1(TRIP) -> Zone2/1
  Zone 4/3(Zr) -> Mux4/2
  Zone 4/2(Zm) -> Mux4/1
  Zone 3/3(Zr) -> Mux3/2
  Zone 3/2(Zm) -> Mux3/1
  Zone 2/3(Zr) -> Mux2/2
  Zone 2/2(Zm) -> Mux2/1
  Zone 1/3(Zr) -> Mux1/2
  Zone 1/2(Zm) -> Mux1/1
  Zone 1/1(TRIP) -> Zone1/1
  Mux/1 -> Zone 2/1(Z), Zone 4/1(Z), Zone 3/1(Z), Zone 1/1(Z)
  C-G/1 -> Voltage Current/1

== system Copy_5_of_baseModel/SM_WT1/Impedance Element 2/Impedance Relay Scheme/Logic Matrix ==
  note: Impedance Relay - Logic Signal Matrix
  A-G : Inport
  B-G : Inport  Port=2
  C-G : Inport  Port=3
  B-C : Inport  Port=4
  C-A : Inport  Port=5
  A-B-C : Inport  Port=6
  A : Logic  Operator=OR  Inputs=3
  A-B-C1 : Logic  Operator=OR  Inputs=4
  "A-G1 " : Logic  Operator=OR  Inputs=4
  B : Logic  Operator=OR  Inputs=3
  B-C1 : Logic  Operator=OR  Inputs=4
  B-G1 : Logic  Operator=OR  Inputs=4
  C : Logic  Operator=OR  Inputs=4
  C-A1 : Logic  Operator=OR  Inputs=4
  C-G1 : Logic  Operator=OR  Inputs=4
  Demux{,1..5} (6 alike) : Demux
  G : Logic  Operator=OR  Inputs=3
  Mux5 : Mux
  zone{1..4} (4 alike) : Logic  Operator=OR  Inputs=6
  " Zone1" : Outport  InitialOutput=0  VectorParamsAs1DForOutWhenUnconnected=on
  " Zone2" : Outport  Port=2  InitialOutput=0  VectorParamsAs1DForOutWhenUnconnected=on
  " Zone3" : Outport  Port=3  InitialOutput=0  VectorParamsAs1DForOutWhenUnconnected=on
  " Zone4" : Outport  Port=4  InitialOutput=0  VectorParamsAs1DForOutWhenUnconnected=on
  Fault Type : Outport  Port=5  InitialOutput=0  VectorParamsAs1DForOutWhenUnconnected=on
  wires:
  G/1 -> Mux5/4
  C/1 -> Mux5/3
  B/1 -> Mux5/2
  A/1 -> Mux5/1
  B-G1/1 -> G/2, B/1
  C-G1/1 -> G/1, C/1
  B-C1/1 -> C/2, B/2
  A-B-C1/1 -> B/3, A/3, C/4
  C-A1/1 -> A/2, C/3
  "A-G1 "/1 -> G/3, A/1
  Demux5/4 -> A-B-C1/4, zone4/6
  Demux5/3 -> A-B-C1/3, zone3/6
  Demux5/2 -> A-B-C1/2, zone2/6
  Demux5/1 -> A-B-C1/1, zone1/6
  Demux4/4 -> C-A1/4, zone4/5
  Demux4/3 -> C-A1/3, zone3/5
  Demux4/2 -> C-A1/2, zone2/5
  Demux4/1 -> C-A1/1, zone1/5
  Demux3/4 -> B-C1/4, zone4/4
  Demux3/3 -> B-C1/3, zone3/4
  Demux3/2 -> B-C1/2, zone2/4
  Demux3/1 -> B-C1/1, zone1/4
  Demux2/4 -> C-G1/4, zone4/3
  Demux2/3 -> C-G1/3, zone3/3
  Demux2/2 -> C-G1/2, zone2/3
  Demux2/1 -> C-G1/1, zone1/3
  Demux1/4 -> B-G1/4, zone4/2
  Demux1/3 -> B-G1/3, zone3/2
  Demux1/2 -> B-G1/2, zone2/2
  Demux1/1 -> B-G1/1, zone1/2
  Demux/4 -> "A-G1 "/4, zone4/1
  Demux/3 -> "A-G1 "/3, zone3/1
  Demux/2 -> "A-G1 "/2, zone2/1
  Demux/1 -> "A-G1 "/1, zone1/1
  A-G/1 -> Demux/1
  B-G/1 -> Demux1/1
  A-B-C/1 -> Demux5/1
  C-A/1 -> Demux4/1
  B-C/1 -> Demux3/1
  C-G/1 -> Demux2/1
  Mux5/1 -> Fault Type/1
  zone1/1 -> " Zone1"/1
  zone2/1 -> " Zone2"/1
  zone4/1 -> " Zone4"/1
  zone3/1 -> " Zone3"/1

== system Copy_5_of_baseModel/SM_WT1/Impedance Element 2/Impedance Relay Scheme/Tripping Logic ==
  note: Impedance Relay - Tripping Logic
  zone1 : Inport
  zone2 : Inport  Port=2
  zone3 : Inport  Port=3
  zone4 : Inport  Port=4
  <V : Inport  Port=5
  Add{,1..3} (4 alike) : Sum
  Constant : Constant  Value=2
  Mux : Mux  Inputs=5
  Mux6 : Mux
  ZM1 + ZM2*t2 + ZM3*t3 + ZM4*t4 : Logic  Operator=OR  Inputs=4
  x2 : Gain  Gain=2  SaturateOnIntegerOverflow=on  OutDataTypeStr=Inherit: Same as input  ParamDataTypeStr=Inherit: Same as input
  x3 : Gain  Gain=3  SaturateOnIntegerOverflow=on  OutDataTypeStr=Inherit: Same as input  ParamDataTypeStr=Inherit: Same as input
  x4 : Gain  Gain=4  SaturateOnIntegerOverflow=on  OutDataTypeStr=Inherit: Same as input  ParamDataTypeStr=Inherit: Same as input
  TRIP : Outport  InitialOutput=0  VectorParamsAs1DForOutWhenUnconnected=on
  Logic Signals : Outport  Port=2  InitialOutput=0  VectorParamsAs1DForOutWhenUnconnected=on
  Fault Zone : Outport  Port=3  InitialOutput=0  VectorParamsAs1DForOutWhenUnconnected=on
  wires:
  Mux6/1 -> Fault Zone/1
  x3/1 -> Add2/2
  x4/1 -> Add3/2
  x2/1 -> Add1/2
  Constant/1 -> x4/1, x3/1, x2/1, Add/2
  Add3/1 -> Mux/5
  Add2/1 -> Mux/4
  Add1/1 -> Mux/3
  Add/1 -> Mux/2
  zone4/1 -> Mux6/4, Add3/1, ZM1 + ZM2*t2 + ZM3*t3 + ZM4*t4/4
  zone3/1 -> Mux6/3, Add2/1, ZM1 + ZM2*t2 + ZM3*t3 + ZM4*t4/3
  zone2/1 -> Add1/1, Mux6/2, ZM1 + ZM2*t2 + ZM3*t3 + ZM4*t4/2
  zone1/1 -> Mux6/1, Add/1, ZM1 + ZM2*t2 + ZM3*t3 + ZM4*t4/1
  ZM1 + ZM2*t2 + ZM3*t3 + ZM4*t4/1 -> TRIP/1
  Mux/1 -> Logic Signals/1
  <V/1 -> Mux/1

== system Copy_5_of_baseModel/SM_WT1/Impedance Element 2/Impedance Relay Scheme/Undervoltage ==
  "Vabc  " : Inport
  Abs : Abs
  Abs1 : Abs
  Abs2 : Abs
  Demux2 : Demux  Outputs=3
  Logical Operator : Logic  Operator=OR  Inputs=3
  Relational Operator : RelationalOperator  Operator=<  RndMeth=Nearest  InputSameDT=on
  Relational Operator1 : RelationalOperator  Operator=<  RndMeth=Nearest  InputSameDT=on
  Relational Operator2 : RelationalOperator  Operator=<  RndMeth=Nearest  InputSameDT=on
  underV Threshold : Constant  Value=underV
  <V : Outport  InitialOutput=0  VectorParamsAs1DForOutWhenUnconnected=on
  wires:
  Demux2/3 -> Abs2/1
  Demux2/2 -> Abs1/1
  Abs1/1 -> Relational Operator2/1
  Abs2/1 -> Relational Operator1/1
  Demux2/1 -> Abs/1
  Abs/1 -> Relational Operator/1
  Relational Operator1/1 -> Logical Operator/3
  Relational Operator/1 -> Logical Operator/1
  Relational Operator2/1 -> Logical Operator/2
  Logical Operator/1 -> <V/1
  underV Threshold/1 -> Relational Operator1/2, Relational Operator2/2, Relational Operator/2
  "Vabc  "/1 -> Demux2/1

== system Copy_5_of_baseModel/SM_WT1/Overcurrent Element 1/Overcurrent Relay Scheme/Analog filtering, signal conditioning ==
  note: Acquisition Block- analog filtering,
      | signal conditioning, sampling.
  Iin : Inport
  CURRENTS : Subsystem
  Mux3 : Mux  Inputs=3
  Mux4 : Mux  Inputs=3
  If : Outport  InitialOutput=0  VectorParamsAs1DForOutWhenUnconnected=on
  If0 : Outport  Port=2  InitialOutput=0  VectorParamsAs1DForOutWhenUnconnected=on
  if : Outport  Port=3  InitialOutput=0  VectorParamsAs1DForOutWhenUnconnected=on
  wires:
  Iin/1 -> CURRENTS/1(Iabc)
  CURRENTS/1(IAf) -> Mux3/1
  CURRENTS/2(IBf) -> Mux3/2
  CURRENTS/3(ICf) -> Mux3/3
  CURRENTS/5(iaf) -> Mux4/1
  CURRENTS/6(ibf) -> Mux4/2
  CURRENTS/7(icf) -> Mux4/3
  Mux3/1 -> If/1
  Mux4/1 -> if/1
  CURRENTS/4(I0f) -> If0/1

== system Copy_5_of_baseModel/SM_WT1/Overcurrent Element 1/Overcurrent Relay Scheme/Logic Matrix ==
  note: Overcurrent Relay - Logic Signal Matrix
  A : Inport
  B : Inport  Port=2
  C : Inport  Port=3
  R : Inport  Port=4
  Mux5 : Mux
  Op : Logic  Operator=OR  Inputs=4
  " Op" : Outport  InitialOutput=0  VectorParamsAs1DForOutWhenUnconnected=on
  Fault Type : Outport  Port=2  InitialOutput=0  VectorParamsAs1DForOutWhenUnconnected=on
  wires:
  Op/1 -> " Op"/1
  Mux5/1 -> Fault Type/1
  R/1 -> Op/4, Mux5/4
  A/1 -> Mux5/1, Op/1
  B/1 -> Mux5/2, Op/2
  C/1 -> Mux5/3, Op/3

== system Copy_5_of_baseModel/SM_WT1/Overcurrent Element 1/Overcurrent Relay Scheme/Phase A ==
  IA : Inport
  Integrator : Integrator
  Operation : Subsystem  mask(Zone){Ip=Iop}
      mask prompts: Ip "PhaseCurrent [A]"
  TRIP output contact : Relay  OnSwitchValue=0.9999  OffSwitchValue=-1
  delay : RelationalOperator  Operator=>  RndMeth=Nearest  InputSameDT=on
  time delay : Constant  Value=Td+0.001
  Pickup : Outport  InitialOutput=0  VectorParamsAs1DForOutWhenUnconnected=on
  wires:
  IA/1 -> Operation/1(Iin)
  Integrator/1 -> delay/1
  time delay/1 -> delay/2
  delay/1 -> TRIP output contact/1
  Operation/1(TRIP) -> Integrator/1
  TRIP output contact/1 -> Pickup/1

== system Copy_5_of_baseModel/SM_WT1/Overcurrent Element 1/Overcurrent Relay Scheme/Phase B ==
  IB : Inport
  Integrator : Integrator
  Operation : Subsystem  mask(Zone){Ip=Iop}
      mask prompts: Ip "PhaseCurrent [A]"
  TRIP output contact : Relay  OnSwitchValue=0.9999  OffSwitchValue=-1
  delay : RelationalOperator  Operator=>  RndMeth=Nearest  InputSameDT=on
  time delay : Constant  Value=Td+0.001
  Pickup : Outport  InitialOutput=0  VectorParamsAs1DForOutWhenUnconnected=on
  wires:
  IB/1 -> Operation/1(Iin)
  Integrator/1 -> delay/1
  time delay/1 -> delay/2
  delay/1 -> TRIP output contact/1
  Operation/1(TRIP) -> Integrator/1
  TRIP output contact/1 -> Pickup/1

== system Copy_5_of_baseModel/SM_WT1/Overcurrent Element 1/Overcurrent Relay Scheme/Phase C ==
  IC : Inport
  Integrator : Integrator
  Operation : Subsystem  mask(Zone){Ip=Iop}
      mask prompts: Ip "PhaseCurrent [A]"
  TRIP output contact : Relay  OnSwitchValue=0.9999  OffSwitchValue=-1
  delay : RelationalOperator  Operator=>  RndMeth=Nearest  InputSameDT=on
  time delay : Constant  Value=Td+0.001
  Pickup : Outport  InitialOutput=0  VectorParamsAs1DForOutWhenUnconnected=on
  wires:
  IC/1 -> Operation/1(Iin)
  Integrator/1 -> delay/1
  time delay/1 -> delay/2
  delay/1 -> TRIP output contact/1
  Operation/1(TRIP) -> Integrator/1
  TRIP output contact/1 -> Pickup/1

== system Copy_5_of_baseModel/SM_WT1/Overcurrent Element 1/Overcurrent Relay Scheme/Residual ==
  IR : Inport
  Integrator : Integrator
  ResCurr : Subsystem  mask(Zone){Ip=ResCurr}
      mask prompts: Ip "PhaseCurrent [A]"
  TRIP output contact : Relay  OnSwitchValue=0.9999  OffSwitchValue=-1  OutDataTypeStr=Inherit: Inherit via back propagation
  delay : RelationalOperator  Operator=>  RndMeth=Nearest  InputSameDT=on
  time delay : Constant  Value=Td+0.001
  Pickup : Outport  InitialOutput=0  VectorParamsAs1DForOutWhenUnconnected=on
  wires:
  IR/1 -> ResCurr/1(Iin)
  Integrator/1 -> delay/1
  time delay/1 -> delay/2
  delay/1 -> TRIP output contact/1
  ResCurr/1(TRIP) -> Integrator/1
  TRIP output contact/1 -> Pickup/1

== system Copy_5_of_baseModel/SM_WT1/Overcurrent Element 1/Overcurrent Relay Scheme/Tripping Logic ==
  note: Overcurrent Relay - Tripping Logic
  Op : Inport
  IR : Inport  Port=2
  Add : Sum
  Constant : Constant  Value=2
  Mux : Mux  Inputs=2
  TRIP : Outport  InitialOutput=0  VectorParamsAs1DForOutWhenUnconnected=on
  Logic Signals : Outport  Port=2  InitialOutput=0  VectorParamsAs1DForOutWhenUnconnected=on
  wires:
  Mux/1 -> Logic Signals/1
  Op/1 -> Add/1, TRIP/1
  Add/1 -> Mux/2
  Constant/1 -> Add/2
  IR/1 -> Mux/1

== system Copy_5_of_baseModel/SM_WT1/Overcurrent Element 2/Overcurrent Relay Scheme/Analog filtering, signal conditioning ==
  note: Acquisition Block- analog filtering,
      | signal conditioning, sampling.
  Iin : Inport
  CURRENTS : Subsystem
  Mux3 : Mux  Inputs=3
  Mux4 : Mux  Inputs=3
  If : Outport  InitialOutput=0  VectorParamsAs1DForOutWhenUnconnected=on
  If0 : Outport  Port=2  InitialOutput=0  VectorParamsAs1DForOutWhenUnconnected=on
  if : Outport  Port=3  InitialOutput=0  VectorParamsAs1DForOutWhenUnconnected=on
  wires:
  Iin/1 -> CURRENTS/1(Iabc)
  CURRENTS/1(IAf) -> Mux3/1
  CURRENTS/2(IBf) -> Mux3/2
  CURRENTS/3(ICf) -> Mux3/3
  CURRENTS/5(iaf) -> Mux4/1
  CURRENTS/6(ibf) -> Mux4/2
  CURRENTS/7(icf) -> Mux4/3
  Mux3/1 -> If/1
  Mux4/1 -> if/1
  CURRENTS/4(I0f) -> If0/1

== system Copy_5_of_baseModel/SM_WT1/Overcurrent Element 2/Overcurrent Relay Scheme/Logic Matrix ==
  note: Overcurrent Relay - Logic Signal Matrix
  A : Inport
  B : Inport  Port=2
  C : Inport  Port=3
  R : Inport  Port=4
  Mux5 : Mux
  Op : Logic  Operator=OR  Inputs=4
  " Op" : Outport  InitialOutput=0  VectorParamsAs1DForOutWhenUnconnected=on
  Fault Type : Outport  Port=2  InitialOutput=0  VectorParamsAs1DForOutWhenUnconnected=on
  wires:
  Op/1 -> " Op"/1
  Mux5/1 -> Fault Type/1
  R/1 -> Op/4, Mux5/4
  A/1 -> Mux5/1, Op/1
  B/1 -> Mux5/2, Op/2
  C/1 -> Mux5/3, Op/3

== system Copy_5_of_baseModel/SM_WT1/Overcurrent Element 2/Overcurrent Relay Scheme/Phase A ==
  IA : Inport
  Integrator : Integrator
  Operation : Subsystem  mask(Zone){Ip=Iop}
      mask prompts: Ip "PhaseCurrent [A]"
  TRIP output contact : Relay  OnSwitchValue=0.9999  OffSwitchValue=-1
  delay : RelationalOperator  Operator=>  RndMeth=Nearest  InputSameDT=on
  time delay : Constant  Value=Td+0.001
  Pickup : Outport  InitialOutput=0  VectorParamsAs1DForOutWhenUnconnected=on
  wires:
  IA/1 -> Operation/1(Iin)
  Integrator/1 -> delay/1
  time delay/1 -> delay/2
  delay/1 -> TRIP output contact/1
  Operation/1(TRIP) -> Integrator/1
  TRIP output contact/1 -> Pickup/1

== system Copy_5_of_baseModel/SM_WT1/Overcurrent Element 2/Overcurrent Relay Scheme/Phase B ==
  IB : Inport
  Integrator : Integrator
  Operation : Subsystem  mask(Zone){Ip=Iop}
      mask prompts: Ip "PhaseCurrent [A]"
  TRIP output contact : Relay  OnSwitchValue=0.9999  OffSwitchValue=-1
  delay : RelationalOperator  Operator=>  RndMeth=Nearest  InputSameDT=on
  time delay : Constant  Value=Td+0.001
  Pickup : Outport  InitialOutput=0  VectorParamsAs1DForOutWhenUnconnected=on
  wires:
  IB/1 -> Operation/1(Iin)
  Integrator/1 -> delay/1
  time delay/1 -> delay/2
  delay/1 -> TRIP output contact/1
  Operation/1(TRIP) -> Integrator/1
  TRIP output contact/1 -> Pickup/1

== system Copy_5_of_baseModel/SM_WT1/Overcurrent Element 2/Overcurrent Relay Scheme/Phase C ==
  IC : Inport
  Integrator : Integrator
  Operation : Subsystem  mask(Zone){Ip=Iop}
      mask prompts: Ip "PhaseCurrent [A]"
  TRIP output contact : Relay  OnSwitchValue=0.9999  OffSwitchValue=-1
  delay : RelationalOperator  Operator=>  RndMeth=Nearest  InputSameDT=on
  time delay : Constant  Value=Td+0.001
  Pickup : Outport  InitialOutput=0  VectorParamsAs1DForOutWhenUnconnected=on
  wires:
  IC/1 -> Operation/1(Iin)
  Integrator/1 -> delay/1
  time delay/1 -> delay/2
  delay/1 -> TRIP output contact/1
  Operation/1(TRIP) -> Integrator/1
  TRIP output contact/1 -> Pickup/1

== system Copy_5_of_baseModel/SM_WT1/Overcurrent Element 2/Overcurrent Relay Scheme/Residual ==
  IR : Inport
  Integrator : Integrator
  ResCurr : Subsystem  mask(Zone){Ip=ResCurr}
      mask prompts: Ip "PhaseCurrent [A]"
  TRIP output contact : Relay  OnSwitchValue=0.9999  OffSwitchValue=-1  OutDataTypeStr=Inherit: Inherit via back propagation
  delay : RelationalOperator  Operator=>  RndMeth=Nearest  InputSameDT=on
  time delay : Constant  Value=Td+0.001
  Pickup : Outport  InitialOutput=0  VectorParamsAs1DForOutWhenUnconnected=on
  wires:
  IR/1 -> ResCurr/1(Iin)
  Integrator/1 -> delay/1
  time delay/1 -> delay/2
  delay/1 -> TRIP output contact/1
  ResCurr/1(TRIP) -> Integrator/1
  TRIP output contact/1 -> Pickup/1

== system Copy_5_of_baseModel/SM_WT1/Overcurrent Element 2/Overcurrent Relay Scheme/Tripping Logic ==
  note: Overcurrent Relay - Tripping Logic
  Op : Inport
  IR : Inport  Port=2
  Add : Sum
  Constant : Constant  Value=2
  Mux : Mux  Inputs=2
  TRIP : Outport  InitialOutput=0  VectorParamsAs1DForOutWhenUnconnected=on
  Logic Signals : Outport  Port=2  InitialOutput=0  VectorParamsAs1DForOutWhenUnconnected=on
  wires:
  Mux/1 -> Logic Signals/1
  Op/1 -> Add/1, TRIP/1
  Add/1 -> Mux/2
  Constant/1 -> Add/2
  IR/1 -> Mux/1

== system Copy_5_of_baseModel/SM_WT1/Overcurrent Inverse time/Overcurrent Relay Scheme/Analog filtering, signal conditioning ==
  note: Acquisition Block- analog filtering,
      | signal conditioning, sampling.
  Iin : Inport
  CURRENTS : Subsystem
  Mux3 : Mux  Inputs=3
  Mux4 : Mux  Inputs=3
  If : Outport  InitialOutput=0  VectorParamsAs1DForOutWhenUnconnected=on
  If0 : Outport  Port=2  InitialOutput=0  VectorParamsAs1DForOutWhenUnconnected=on
  if : Outport  Port=3  InitialOutput=0  VectorParamsAs1DForOutWhenUnconnected=on
  wires:
  Iin/1 -> CURRENTS/1(Iabc)
  CURRENTS/1(IAf) -> Mux3/1
  CURRENTS/2(IBf) -> Mux3/2
  CURRENTS/3(ICf) -> Mux3/3
  CURRENTS/5(iaf) -> Mux4/1
  CURRENTS/6(ibf) -> Mux4/2
  CURRENTS/7(icf) -> Mux4/3
  Mux3/1 -> If/1
  Mux4/1 -> if/1
  CURRENTS/4(I0f) -> If0/1

== system Copy_5_of_baseModel/SM_WT1/Overcurrent Inverse time/Overcurrent Relay Scheme/Logic Matrix ==
  note: Overcurrent Relay - Logic Signal Matrix
  A : Inport
  B : Inport  Port=2
  C : Inport  Port=3
  Mux5 : Mux  Inputs=3
  Op : Logic  Operator=OR  Inputs=3
  " Op" : Outport  InitialOutput=0  VectorParamsAs1DForOutWhenUnconnected=on
  Fault Type : Outport  Port=2  InitialOutput=0  VectorParamsAs1DForOutWhenUnconnected=on
  wires:
  Op/1 -> " Op"/1
  Mux5/1 -> Fault Type/1
  A/1 -> Mux5/1, Op/1
  B/1 -> Mux5/2, Op/2
  C/1 -> Mux5/3, Op/3

== system Copy_5_of_baseModel/SM_WT1/Overcurrent Inverse time/Overcurrent Relay Scheme/Phase A ==
  IA : Inport
  Integrator : Integrator
  Operation : Subsystem  mask(Zone){Ip=Iop}
      mask prompts: Ip "PhaseCurrent [A]"
  Subsystem : Subsystem
  TRIP output contact : Relay  OnSwitchValue=0.9999  OffSwitchValue=-1
  delay : RelationalOperator  Operator=>  RndMeth=Nearest  InputSameDT=on
  Pickup : Outport  InitialOutput=0  VectorParamsAs1DForOutWhenUnconnected=on
  wires:
  Operation/1(TRIP) -> Integrator/1
  TRIP output contact/1 -> Pickup/1
  IA/1 -> Operation/1(Iin), Subsystem/1("Current ")
  delay/1 -> TRIP output contact/1
  Integrator/1 -> delay/1
  Subsystem/1(Time) -> delay/2

== system Copy_5_of_baseModel/SM_WT1/Overcurrent Inverse time/Overcurrent Relay Scheme/Phase B ==
  IB : Inport
  Integrator : Integrator
  Operation : Subsystem  mask(Zone){Ip=Iop}
      mask prompts: Ip "PhaseCurrent [A]"
  Subsystem : Subsystem
  TRIP output contact : Relay  OnSwitchValue=0.9999  OffSwitchValue=-1
  delay : RelationalOperator  Operator=>  RndMeth=Nearest  InputSameDT=on
  Pickup : Outport  InitialOutput=0  VectorParamsAs1DForOutWhenUnconnected=on
  wires:
  Integrator/1 -> delay/1
  Subsystem/1(Time) -> delay/2
  Operation/1(TRIP) -> Integrator/1
  IB/1 -> Operation/1(Iin), Subsystem/1("Current ")
  delay/1 -> TRIP output contact/1
  TRIP output contact/1 -> Pickup/1

== system Copy_5_of_baseModel/SM_WT1/Overcurrent Inverse time/Overcurrent Relay Scheme/Phase C ==
  IC : Inport
  Integrator2 : Integrator
  Operation1 : Subsystem  mask(Zone){Ip=Iop}
      mask prompts: Ip "PhaseCurrent [A]"
  Subsystem1 : Subsystem
  TRIP output contact1 : Relay  OnSwitchValue=0.9999  OffSwitchValue=-1
  delay2 : RelationalOperator  Operator=>  RndMeth=Nearest  InputSameDT=on
  Pickup : Outport  InitialOutput=0  VectorParamsAs1DForOutWhenUnconnected=on
  wires:
  Integrator2/1 -> delay2/1
  Subsystem1/1(Time) -> delay2/2
  Operation1/1(TRIP) -> Integrator2/1
  IC/1 -> Subsystem1/1("Current "), Operation1/1(Iin)
  delay2/1 -> TRIP output contact1/1
  TRIP output contact1/1 -> Pickup/1

== system Copy_5_of_baseModel/SM_WT1/Overcurrent Inverse time/Overcurrent Relay Scheme/Tripping Logic ==
  note: Overcurrent Relay - Tripping Logic
  Op : Inport
  TRIP : Outport  InitialOutput=0  VectorParamsAs1DForOutWhenUnconnected=on
  wires:
  Op/1 -> TRIP/1
